simulink model "proy"  (R2022b)
settings: Solver=VariableStepAuto  StartTime=0.0  StopTime=24  RelTol=1e-3
model workspace (MAT data in the model file):
  M_aire_calentador = 3600
  M_aire_casa = 1470
  R_equiv = 4.329e-07
  TCasa_IC = 20
  c_aire = 1005.4
  temp_C = 50
settings Model: Creator=ec0822  LastModifiedBy=ec0822

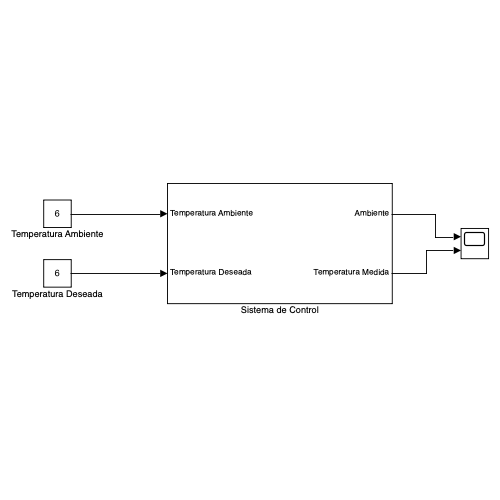
[thumbnail: Simulink's stored preview of the top-level diagram]
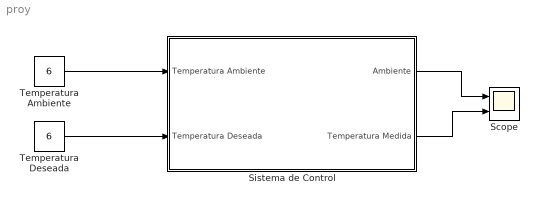
== system proy ==
  Scope : Scope  NumInputPorts=2
  Sistema de Control : Subsystem
  Temperatura Ambiente : Constant  Value=6
  Temperatura Deseada : Constant  Value=6
  wires:
  Temperatura Ambiente/1 -> Sistema de Control/1(Temperatura Ambiente)
  Temperatura Deseada/1 -> Sistema de Control/2(Temperatura Deseada)
  Sistema de Control/1(Ambiente) -> Scope/1
  Sistema de Control/2(Temperatura Medida) -> Scope/2

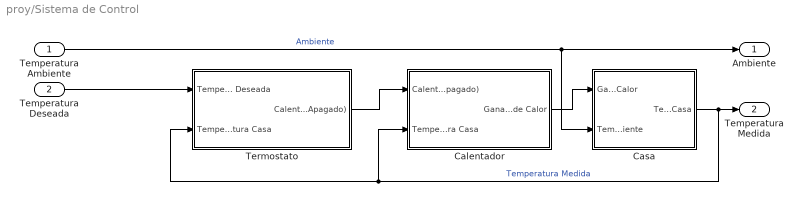
== system proy/Sistema de Control ==
  Temperatura Ambiente : Inport
  Temperatura Deseada : Inport  Port=2
  Calentador : Subsystem
  Casa : Subsystem
  Termostato : Subsystem
  Ambiente : Outport
  Temperatura Medida : Outport  Port=2
  wires:
  Termostato/1(Calentador (Encendido/Apagado)) -> Calentador/1(Calentador (Encendido/Apagado))
  Calentador/1(Ganancia de Calor) -> Casa/1(Ganancia de Calor)
  Casa/1(Temperatura Casa) -> Temperatura Medida/1, Termostato/2(Temperatura Casa), Calentador/2(Temperatura Casa)  "Temperatura Medida"
  Temperatura Deseada/1 -> Termostato/1(Temperatura Deseada)
  Temperatura Ambiente/1 -> Ambiente/1, Casa/2(Temperatura Ambiente)  "Ambiente"

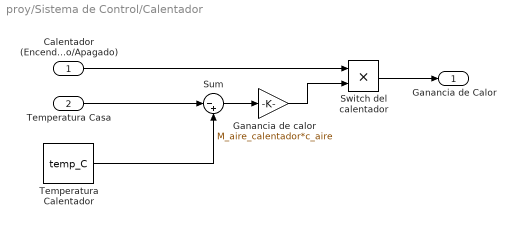
== system proy/Sistema de Control/Calentador ==
  Calentador (Encendido/Apagado) : Inport
  Temperatura Casa : Inport  Port=2
  Ganancia de calor : Gain  Gain=M_aire_calentador*c_aire
  Sum : Sum  Inputs=|-+
  Switch del calentador : Product
  Temperatura Calentador : Constant  Value=temp_C
  Ganancia de Calor : Outport
  wires:
  Calentador (Encendido/Apagado)/1 -> Switch del calentador/1
  Temperatura Casa/1 -> Sum/1
  Temperatura Calentador/1 -> Sum/2
  Sum/1 -> Ganancia de calor/1
  Ganancia de calor/1 -> Switch del calentador/2
  Switch del calentador/1 -> Ganancia de Calor/1

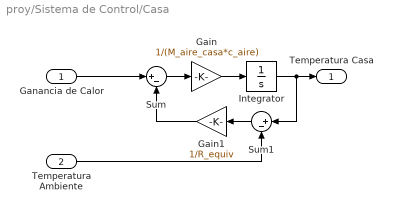
== system proy/Sistema de Control/Casa ==
  Ganancia de Calor : Inport
  Temperatura Ambiente : Inport  Port=2
  Gain : Gain  Gain=1/(M_aire_casa*c_aire)
  Gain1 : Gain  Gain=1/R_equiv
  Integrator : Integrator  InitialCondition=TCasa_IC
  Sum : Sum  Inputs=|+-
  Sum1 : Sum  Inputs=|+-
  Temperatura Casa : Outport
  wires:
  Gain/1 -> Integrator/1
  Sum1/1 -> Gain1/1
  Integrator/1 -> Sum1/1, Temperatura Casa/1
  Temperatura Ambiente/1 -> Sum1/2
  Gain1/1 -> Sum/2
  Sum/1 -> Gain/1
  Ganancia de Calor/1 -> Sum/1

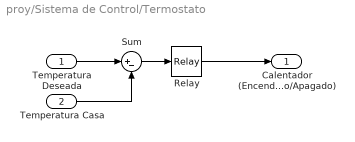
== system proy/Sistema de Control/Termostato ==
  Temperatura Deseada : Inport
  Temperatura Casa : Inport  Port=2
  Relay : Relay  OnSwitchValue=2  OffSwitchValue=-2
  Sum : Sum  Inputs=|+-
  Calentador (Encendido/Apagado) : Outport
  wires:
  Temperatura Deseada/1 -> Sum/1
  Temperatura Casa/1 -> Sum/2
  Sum/1 -> Relay/1
  Relay/1 -> Calentador (Encendido/Apagado)/1
